simulink model "OASIS"  (R2024b)
settings: Solver=ode3  StartTime=0.0  StopTime=86400  FixedStep=1  MaxStep=0.1  RelTol=1e-3
PostLoadFcn:
  | init_OASIS
InitFcn:
  | init_OASIS
values from neighbouring files (symbols this model uses):
  DiscreteON = 1    [init_OASIS.m]
  GridON = 1    [init_OASIS.m]
  P_cargador_EV = 50000    [init_OASIS.m]
undefined symbols (not defined in the file or in its folder): DiscIntNeverNeededParam, Tamb
(part 3 of 3)

== system OASIS/Cuadro de Control 2 ==
  note: Battery
  note: Manual Mode
  note: Manual Power Ref. (kW)
  note: Power (kW)
  note: Charge
  note: Discharge
  note: State of Charge
  note: Voltage
  note: Current
  Dashboard Scope : DashboardScope  Ymin=-2000  Ymax=2000  LegendPosition=Hide  ScaleAtStop=off
  Dashboard Scope1 : DashboardScope  Ymin=0  Ymax=100  LegendPosition=Hide  ScaleAtStop=off
  Gauge : CircularGaugeBlock  LabelPosition=Hide  ScaleMax=450
  Gauge1 : CircularGaugeBlock  LabelPosition=Hide  ScaleMin=-5000  ScaleMax=5000  TickInterval=1000
  Slider : SliderBlock  LabelPosition=Hide  ScaleMin=-2000  ScaleMax=2000
  Toggle Switch : ToggleSwitchBlock  LabelPosition=Hide
      settings: Values={{'Off', 'On'}, [0 1]}

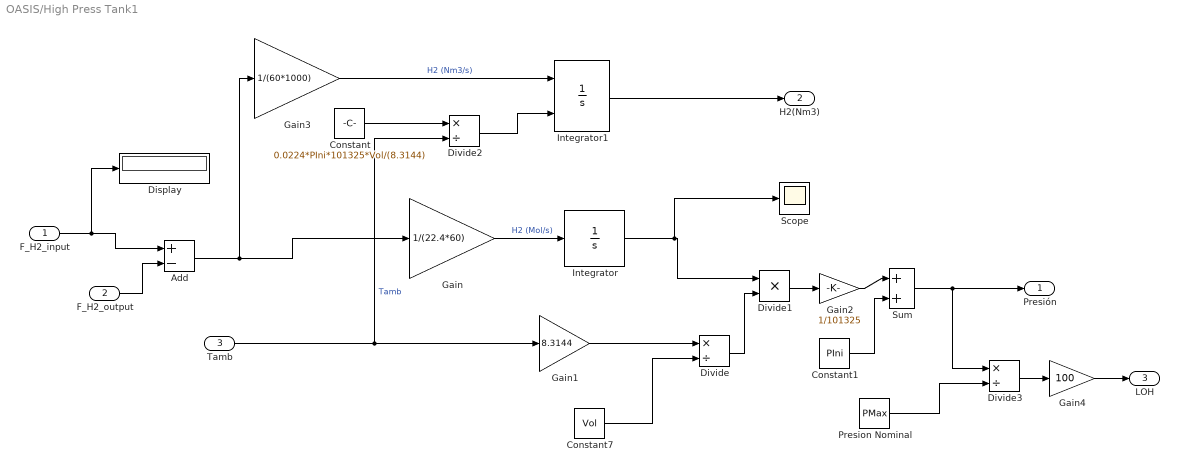
== system OASIS/High Press Tank1 ==
  F_H2_input : Inport
  F_H2_output : Inport  Port=2
  Tamb : Inport  Port=3
  Add : Sum  Inputs=+-
  Constant : Constant  Value=0.0224*PIni*101325*Vol/(8.3144)
  Constant1 : Constant  Value=PIni
  Constant7 : Constant  Value=Vol
  Display : Display
  Divide : Product  Inputs=*/
  Divide1 : Product  Inputs=**
  Divide2 : Product  Inputs=*/
  Divide3 : Product  Inputs=*/
  Gain : Gain  Gain=1/(22.4*60)
  Gain1 : Gain  Gain=8.3144
  Gain2 : Gain  Gain=1/101325
  Gain3 : Gain  Gain=1/(60*1000)
  Gain4 : Gain  Gain=100
  Integrator : Integrator
  Integrator1 : Integrator  InitialConditionSource=external  InitialCondition=PIni*101325*Vol/(8.3144*Tamb*1000)
  Presion Nominal : Constant  Value=PMax
  Scope : Scope
  Sum : Sum  Inputs=|++
  Presión : Outport
  H2(Nm3) : Outport  Port=2
  LOH : Outport  Port=3
  wires:
  Integrator/1 -> Scope/1, Divide1/1
  Divide1/1 -> Gain2/1
  Constant7/1 -> Divide/2
  Gain/1 -> Integrator/1  "H2 (Mol/s)"
  Tamb/1 -> Divide2/2, Gain1/1  "Tamb"
  Gain1/1 -> Divide/1
  Divide/1 -> Divide1/2
  Integrator1/1 -> H2(Nm3)/1
  Gain3/1 -> Integrator1/1  "H2 (Nm3/s)"
  Sum/1 -> Divide3/1, Presión/1
  Gain2/1 -> Sum/1
  Constant1/1 -> Sum/2
  Constant/1 -> Divide2/1
  Divide2/1 -> Integrator1/2
  Add/1 -> Gain3/1, Gain/1
  F_H2_input/1 -> Display/1, Add/1
  F_H2_output/1 -> Add/2
  Presion Nominal/1 -> Divide3/2
  Divide3/1 -> Gain4/1
  Gain4/1 -> LOH/1

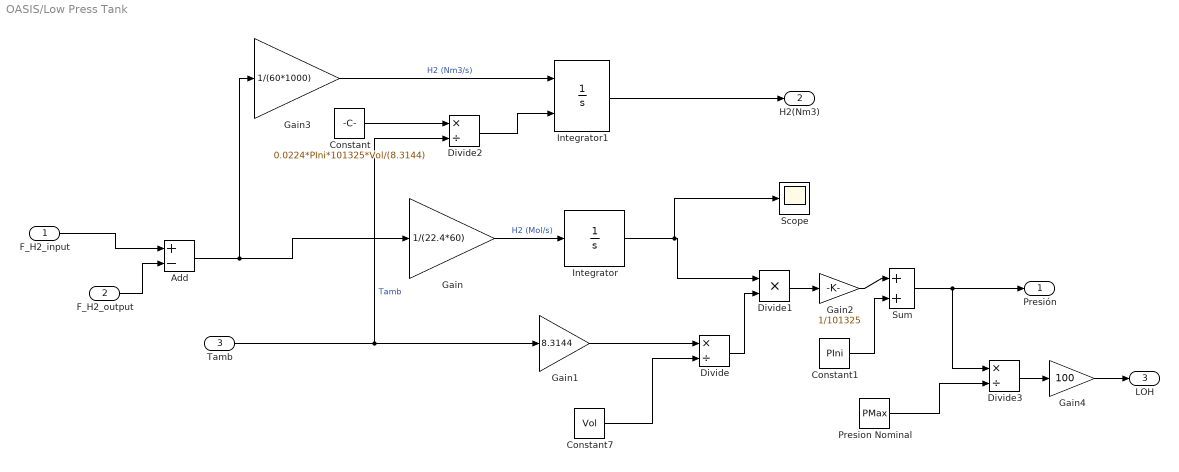
== system OASIS/Low Press Tank ==
  F_H2_input : Inport
  F_H2_output : Inport  Port=2
  Tamb : Inport  Port=3
  Add : Sum  Inputs=+-
  Constant : Constant  Value=0.0224*PIni*101325*Vol/(8.3144)
  Constant1 : Constant  Value=PIni
  Constant7 : Constant  Value=Vol
  Divide : Product  Inputs=*/
  Divide1 : Product  Inputs=**
  Divide2 : Product  Inputs=*/
  Divide3 : Product  Inputs=*/
  Gain : Gain  Gain=1/(22.4*60)
  Gain1 : Gain  Gain=8.3144
  Gain2 : Gain  Gain=1/101325
  Gain3 : Gain  Gain=1/(60*1000)
  Gain4 : Gain  Gain=100
  Integrator : Integrator
  Integrator1 : Integrator  InitialConditionSource=external  InitialCondition=PIni*101325*Vol/(8.3144*Tamb*1000)
  Presion Nominal : Constant  Value=PMax
  Scope : Scope
  Sum : Sum  Inputs=|++
  Presión : Outport
  H2(Nm3) : Outport  Port=2
  LOH : Outport  Port=3
  wires:
  Integrator/1 -> Scope/1, Divide1/1
  Divide1/1 -> Gain2/1
  Constant7/1 -> Divide/2
  Gain/1 -> Integrator/1  "H2 (Mol/s)"
  Tamb/1 -> Divide2/2, Gain1/1  "Tamb"
  Gain1/1 -> Divide/1
  Divide/1 -> Divide1/2
  Integrator1/1 -> H2(Nm3)/1
  Gain3/1 -> Integrator1/1  "H2 (Nm3/s)"
  Sum/1 -> Divide3/1, Presión/1
  Gain2/1 -> Sum/1
  Constant1/1 -> Sum/2
  Constant/1 -> Divide2/1
  Divide2/1 -> Integrator1/2
  Add/1 -> Gain3/1, Gain/1
  F_H2_input/1 -> Add/1
  F_H2_output/1 -> Add/2
  Presion Nominal/1 -> Divide3/2
  Divide3/1 -> Gain4/1
  Gain4/1 -> LOH/1

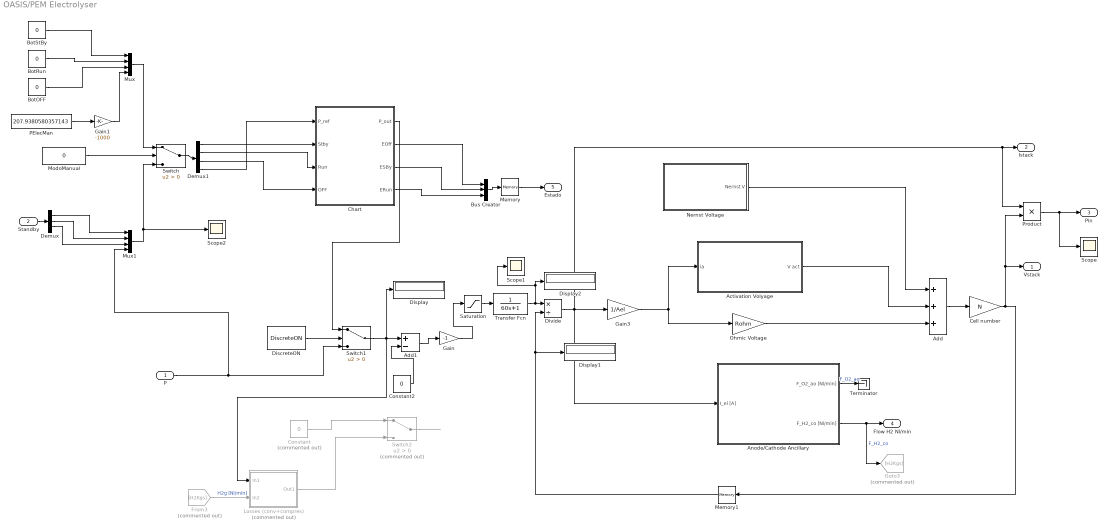
== system OASIS/PEM Electrolyser ==
  P : Inport
  Standby : Inport  Port=2
  Activation Volyage : Subsystem
  Add : Sum  Inputs=+++
  Add1 : Sum  Inputs=+-
  Anode/Cathode Ancillary : Subsystem
  BotOFF : Constant  Value=0
  BotRun : Constant  Value=0
  BotStBy : Constant  Value=0
  Bus Creator : BusCreator  Inputs=3
  Cell number : Gain  Gain=N
  Chart : Stateflow chart  TreatAsAtomicUnit=on
  Constant : Constant  Commented=on  Value=0
  Constant2 : Constant  Value=0
  Demux : Demux  Outputs=3
  Demux1 : Demux
  DiscreteON : Constant  Value=DiscreteON
  Display : Display
  Display1 : Display
  Display2 : Display
  Divide : Product  Inputs=*/
  From3 : From  Commented=on  GotoTag=H2Kgs
  Gain : Gain  Gain=-1
  Gain1 : Gain  Gain=-1000
  Gain3 : Gain  Gain=1/Ael
  Goto3 : Goto  Commented=on  GotoTag=H2Kgs
  Losses (conv+compres) : Subsystem  Commented=on
  Memory : Memory
  Memory1 : Memory  InitialCondition=115
  ModoManual : Constant  Value=0
  Mux : Mux
  Mux1 : Mux
  Nernst Voltage : Subsystem
  Ohmic Voltage : Gain  Gain=Rohm
  PElecMan : Constant  Value=207.9380580357143
  Product : Product
  Saturation : Saturate  UpperLimit=Pmax  LowerLimit=0
  Scope : Scope
  Scope1 : Scope
  Scope2 : Scope
  Switch : Switch  Criteria=u2 > Threshold  SaturateOnIntegerOverflow=off  InputSameDT=off
  Switch1 : Switch  Criteria=u2 > Threshold  SaturateOnIntegerOverflow=off  InputSameDT=off
  Switch2 : Switch  Commented=on  Criteria=u2 > Threshold  SaturateOnIntegerOverflow=off  InputSameDT=off
  Terminator : Terminator
  Transfer Fcn : TransferFcn  Denominator=[60 1]
  Vstack : Outport  VectorParamsAs1DForOutWhenUnconnected=off
  Istack : Outport  Port=2  VectorParamsAs1DForOutWhenUnconnected=off
  Pin : Outport  Port=3  VectorParamsAs1DForOutWhenUnconnected=off
  "Flow H2 Nl/min " : Outport  Port=4  VectorParamsAs1DForOutWhenUnconnected=off
  Estado : Outport  Port=5  VectorParamsAs1DForOutWhenUnconnected=off
  wires:
  Product/1 -> Scope/1, Pin/1
  Gain/1 -> Saturation/1
  Ohmic Voltage/1 -> Add/3
  Activation Volyage/1(V act) -> Add/2
  Cell number/1 -> Memory1/1, Vstack/1, Product/2
  Nernst Voltage/1(Nernst V) -> Add/1
  Add/1 -> Cell number/1
  Divide/1 -> Gain3/1, Istack/1, Product/1, Anode/Cathode Ancillary/1(I_el [A])
  Memory1/1 -> Display1/1, Divide/2
  Gain3/1 -> Ohmic Voltage/1, Activation Volyage/1(ia)
  Anode/Cathode Ancillary/2(F_H2_co [Nl/min]) -> Goto3/1, "Flow H2 Nl/min "/1  "F_H2_co"
  ModoManual/1 -> Switch/2
  PElecMan/1 -> Gain1/1
  P/1 -> Mux1/4, Switch1/3
  Chart/1(P_out) -> Switch1/1
  Saturation/1 -> Transfer Fcn/1
  Transfer Fcn/1 -> Scope1/1, Display2/1, Divide/1
  DiscreteON/1 -> Switch1/2
  Add1/1 -> Gain/1
  Switch1/1 -> Display/1, Add1/1, Losses (conv+compres)/1(In1)
  Constant/1 -> Switch2/1
  Losses (conv+compres)/1(Out1) -> Switch2/3
  From3/1 -> Losses (conv+compres)/2(In2)  "H2g [Nl/min]"
  Bus Creator/1 -> Memory/1
  Memory/1 -> Estado/1
  BotStBy/1 -> Mux/1
  BotRun/1 -> Mux/2
  BotOFF/1 -> Mux/3
  Gain1/1 -> Mux/4
  Mux/1 -> Switch/1
  Switch/1 -> Demux1/1
  Demux1/1 -> Chart/2(Stby)
  Demux1/2 -> Chart/3(Run)
  Demux1/3 -> Chart/4(OFF)
  Demux1/4 -> Chart/1(P_ref)
  Standby/1 -> Demux/1
  Demux/1 -> Mux1/1
  Demux/2 -> Mux1/2
  Mux1/1 -> Scope2/1, Switch/3
  Demux/3 -> Mux1/3
  Chart/2(EOff) -> Bus Creator/1
  Chart/3(ESBy) -> Bus Creator/2
  Chart/4(ERun) -> Bus Creator/3
  Constant2/1 -> Add1/2
  Anode/Cathode Ancillary/1(F_O2_ao [Nl/min]) -> Terminator/1  "F_O2_ao"
  Switch2/1 -> ?

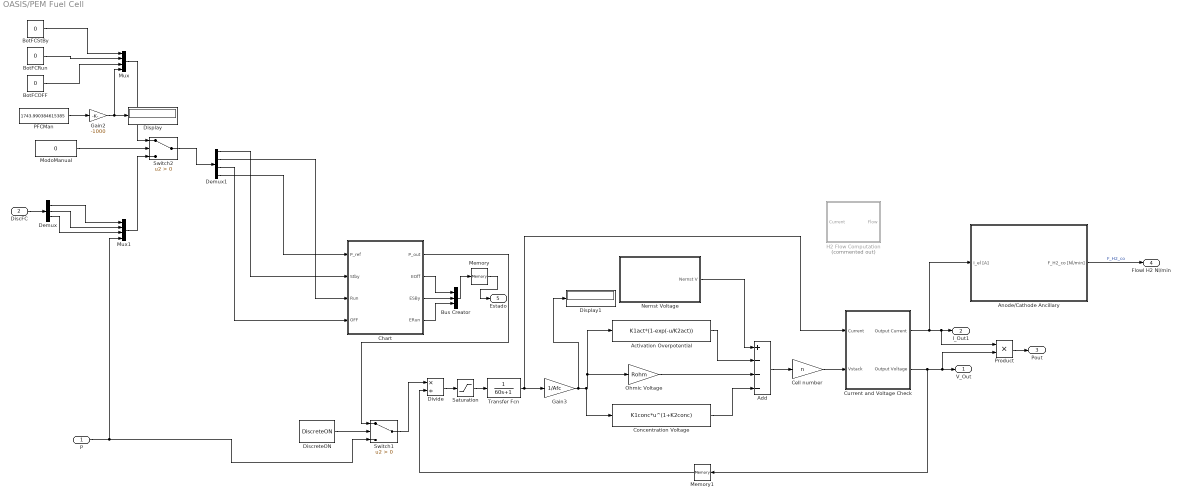
== system OASIS/PEM Fuel Cell ==
  P : Inport
  DiscFC : Inport  Port=2
  "Activation Overpotential " : Fcn  Expr=K1act*(1-exp(-u/K2act))
  Add : Sum  Inputs=+---
  Anode/Cathode Ancillary : Subsystem
  BotFCOFF : Constant  Value=0
  BotFCRun : Constant  Value=0
  BotFCStBy : Constant  Value=0
  Bus Creator : BusCreator  Inputs=3
  Cell number : Gain  Gain=n
  Chart : Stateflow chart  TreatAsAtomicUnit=on
  Concentration Voltage : Fcn  Expr=K1conc*u^(1+K2conc)
  Current and Voltage Check : Subsystem
  Demux : Demux  Outputs=3
  Demux1 : Demux
  DiscreteON : Constant  Value=DiscreteON
  Display : Display
  Display1 : Display
  Divide : Product  Inputs=*/
  Gain2 : Gain  Gain=-1000
  Gain3 : Gain  Gain=1/Afc
  H2 Flow Computation : Subsystem  Commented=on
  Memory : Memory
  Memory1 : Memory  InitialCondition=600
  ModoManual : Constant  Value=0
  Mux : Mux
  Mux1 : Mux
  Nernst Voltage : Subsystem
  Ohmic Voltage : Gain  Gain=Rohm
  PFCMan : Constant  Value=1743.990384615385
  Product : Product
  Saturation : Saturate  UpperLimit=Imax  LowerLimit=0
  Switch1 : Switch  Criteria=u2 > Threshold  SaturateOnIntegerOverflow=off  InputSameDT=off
  Switch2 : Switch  Criteria=u2 > Threshold  SaturateOnIntegerOverflow=off  InputSameDT=off
  Transfer Fcn : TransferFcn  Denominator=[60 1]
  V_Out : Outport  VectorParamsAs1DForOutWhenUnconnected=off
  I_Out1 : Outport  Port=2  VectorParamsAs1DForOutWhenUnconnected=off
  Pout : Outport  Port=3  VectorParamsAs1DForOutWhenUnconnected=off
  Flowl H2 Nl/min : Outport  Port=4  VectorParamsAs1DForOutWhenUnconnected=off
  Estado : Outport  Port=5  VectorParamsAs1DForOutWhenUnconnected=off
  wires:
  Product/1 -> Pout/1
  Cell number/1 -> Current and Voltage Check/2(Vstack)
  Divide/1 -> Saturation/1
  Current and Voltage Check/1(Output Current) -> Anode/Cathode Ancillary/1(I_el [A]), I_Out1/1, Product/1
  Current and Voltage Check/2(Output Voltage) -> V_Out/1, Product/2, Memory1/1
  "Activation Overpotential "/1 -> Add/2
  Nernst Voltage/1(Nernst V) -> Add/1
  Gain3/1 -> Display1/1, Ohmic Voltage/1, "Activation Overpotential "/1, Concentration Voltage/1
  Ohmic Voltage/1 -> Add/3
  Memory1/1 -> Divide/2
  Add/1 -> Cell number/1
  Anode/Cathode Ancillary/1(F_H2_co [Nl/min]) -> Flowl H2 Nl/min/1  "F_H2_co"
  Concentration Voltage/1 -> Add/4
  Saturation/1 -> Transfer Fcn/1
  Chart/3(ESBy) -> Bus Creator/2
  Chart/4(ERun) -> Bus Creator/3
  Chart/2(EOff) -> Bus Creator/1
  Transfer Fcn/1 -> Current and Voltage Check/1(Current), Gain3/1
  DiscreteON/1 -> Switch1/2
  Chart/1(P_out) -> Switch1/1
  Switch1/1 -> Divide/1
  Bus Creator/1 -> Memory/1
  Demux/3 -> Mux1/3
  DiscFC/1 -> Demux/1
  BotFCRun/1 -> Mux/2
  Demux/2 -> Mux1/2
  Demux/1 -> Mux1/1
  BotFCOFF/1 -> Mux/3
  Gain2/1 -> Mux/4, Display/1
  P/1 -> Switch1/3, Mux1/4
  ModoManual/1 -> Switch2/2
  Mux/1 -> Switch2/1
  BotFCStBy/1 -> Mux/1
  Mux1/1 -> Switch2/3
  PFCMan/1 -> Gain2/1
  Switch2/1 -> Demux1/1
  Memory/1 -> Estado/1
  Demux1/4 -> Chart/1(P_ref)
  Demux1/1 -> Chart/2(Stby)
  Demux1/2 -> Chart/3(Run)
  Demux1/3 -> Chart/4(OFF)

== system OASIS/Predicciones LSTM ==
  Clock1 : Clock
  From Workspace1 : FromWorkspace  VariableName=features_solar  SampleTime=900
  From Workspace2 : FromWorkspace  VariableName=dia_anno  SampleTime=1
  From Workspace3 : FromWorkspace  VariableName=features_precio  SampleTime=1
  From Workspace4 : FromWorkspace  VariableName=dia_semana  SampleTime=1
  Gain4 : Gain  Gain=490
  Modelo LSTM Irradianza : M-S-Function  FunctionName=lstm_sol
  Modelo LSTM Precio : M-S-Function  FunctionName=lstm_precios
  W : Outport
  €/MW : Outport  Port=2
  W/m2 : Outport  Port=3
  wires:
  Clock1/1 -> Modelo LSTM Precio/2, Modelo LSTM Irradianza/2
  Gain4/1 -> W/1  "W"
  Modelo LSTM Precio/1 -> €/MW/1  "€/MW"
  From Workspace3/1 -> Modelo LSTM Precio/1
  Modelo LSTM Irradianza/1 -> W/m2/1, Gain4/1  "W/m2"
  From Workspace1/1 -> Modelo LSTM Irradianza/1
  From Workspace2/1 -> Modelo LSTM Precio/3
  From Workspace4/1 -> Modelo LSTM Precio/4

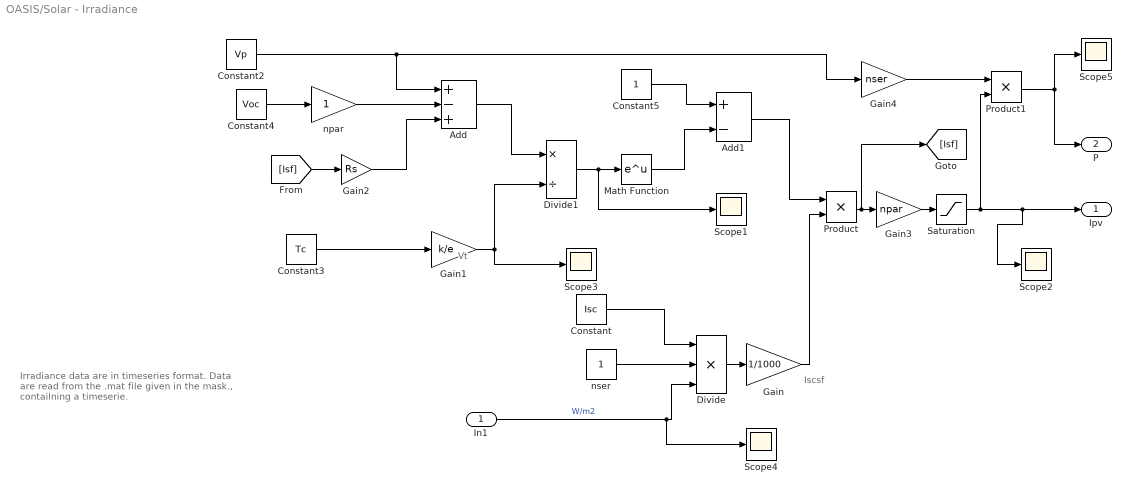
== system OASIS/Solar - Irradiance ==
  note: Vt
  note: Iscsf
  note: Irradiance data are in timeseries format.
      |
      | Data are read from the .mat file given in the mask., contailning a timeserie.
  In1 : Inport
  Add : Sum  Inputs=+-+
  Add1 : Sum  Inputs=+-
  Constant : Constant  Value=Isc
  Constant2 : Constant  Value=Vp
  Constant3 : Constant  Value=Tc
  Constant4 : Constant  Value=Voc
  Constant5 : Constant
  Divide : Product  Inputs=***
  Divide1 : Product  Inputs=*/
  Gain : Gain  Gain=1/1000
  Gain1 : Gain  Gain=k/e
  Gain2 : Gain  Gain=Rs
  Gain3 : Gain  Gain=npar
  Gain4 : Gain  Gain=nser
  Math Function : Math  SignedPower=on
  Product : Product
  Product1 : Product
  Saturation : Saturate  UpperLimit=inf  LowerLimit=0
  Scope{1..5} (5 alike) : Scope
  npar : Gain
  nser : Constant
  Ipv : Outport  VectorParamsAs1DForOutWhenUnconnected=off
  P : Outport  Port=2  VectorParamsAs1DForOutWhenUnconnected=off
  wires:
  Constant/1 -> Divide/1
  nser/1 -> Divide/2
  Divide/1 -> Gain/1
  Gain/1 -> Product/2
  Gain1/1 -> Scope3/1, Divide1/2
  Constant2/1 -> Gain4/1, Add/1
  Constant4/1 -> npar/1
  [Isf] -> Gain2/1
  Gain2/1 -> Add/3
  Divide1/1 -> Scope1/1, Math Function/1
  Math Function/1 -> Add1/2
  Constant5/1 -> Add1/1
  Add1/1 -> Product/1
  Add/1 -> Divide1/1
  Saturation/1 -> Product1/2, Scope2/1, Ipv/1
  Constant3/1 -> Gain1/1
  npar/1 -> Add/2
  Product1/1 -> Scope5/1, P/1
  In1/1 -> Scope4/1, Divide/3  "W/m2"
  Gain4/1 -> Product1/1
  Product/1 -> [Isf], Gain3/1
  Gain3/1 -> Saturation/1

== system OASIS/Subsystem2 ==

== system OASIS/Subsystem3 ==

== system OASIS/Battery/Charge ==
  Intensidad : Inport
  IntegralI : Inport  Port=2
  Fcn1 : Fcn  Expr=Kbt*C120bt/(C120bt+0.1*u)
  Product : Product
  Out1 : Outport  VectorParamsAs1DForOutWhenUnconnected=off
  wires:
  Fcn1/1 -> Product/2
  Product/1 -> Out1/1
  Intensidad/1 -> Product/1
  IntegralI/1 -> Fcn1/1

== system OASIS/Battery/Discharge ==
  Intensidad : Inport
  IntegralI : Inport  Port=2
  Fcn1 : Fcn  Expr=Kbt*C120bt/((C120bt-u))
  Product : Product
  Out1 : Outport  VectorParamsAs1DForOutWhenUnconnected=off
  wires:
  Intensidad/1 -> Product/1
  Product/1 -> Out1/1
  Fcn1/1 -> Product/2
  IntegralI/1 -> Fcn1/1

== system OASIS/Battery/SOC Computation ==
  In1 : Inport
  Add3 : Sum  Inputs=+-
  C120,bt2 : Constant  Value=C120bt
  Divide2 : Product  Inputs=/*
  Gain6 : Gain  Gain=100
  Out1 : Outport  VectorParamsAs1DForOutWhenUnconnected=off
  wires:
  Add3/1 -> Gain6/1
  In1/1 -> Add3/2
  Gain6/1 -> Divide2/2
  C120,bt2/1 -> Divide2/1, Add3/1
  Divide2/1 -> Out1/1

== system OASIS/Battery/SOC=100 or SOC=0 ==
  ISOC : Inport
  P : Inport  Port=2
  Constant : Constant  Value=100
  Constant1 : Constant  Value=0
  Constant2 : Constant  Value=0
  Gain2 : Gain  Gain=-1
  Logical Operator : Logic  AllPortsSameDT=off  OutDataTypeStr=boolean
  Logical Operator1 : Logic  Operator=OR  AllPortsSameDT=off  OutDataTypeStr=boolean
  Product : Product
  Relational Operator : RelationalOperator  OutDataTypeStr=boolean  InputSameDT=off
  Relational Operator1 : RelationalOperator  Operator=<=  OutDataTypeStr=boolean  InputSameDT=off
  Relational Operator2 : RelationalOperator  OutDataTypeStr=boolean  InputSameDT=off
  Sign : Signum
  Out1 : Outport  VectorParamsAs1DForOutWhenUnconnected=off
  wires:
  P/1 -> Sign/1
  Sign/1 -> Relational Operator2/1, Product/2
  ISOC/1 -> Relational Operator1/1, Product/1
  Product/1 -> Gain2/1
  Gain2/1 -> Relational Operator/1
  Constant/1 -> Relational Operator/2
  Constant1/1 -> Relational Operator1/2
  Constant2/1 -> Relational Operator2/2
  Relational Operator2/1 -> Logical Operator/1
  Relational Operator1/1 -> Logical Operator/2
  Logical Operator1/1 -> Out1/1
  Relational Operator/1 -> Logical Operator1/1
  Logical Operator/1 -> Logical Operator1/2

== system OASIS/PEM Electrolyser/Activation Volyage ==
  ia : Inport
  Add1 : Sum
  Gain : Gain  Gain=R*Tel/F
  Gain1 : Gain  Gain=0.5/iao
  Gain2 : Gain  Gain=0.5/ico
  "asinh " : Fcn  Expr=log(u+sqrt(u*u+1))
  asinh 1 : Fcn  Expr=log(u+sqrt(u*u+1))
  V act : Outport  VectorParamsAs1DForOutWhenUnconnected=off
  wires:
  Gain1/1 -> "asinh "/1
  ia/1 -> Gain2/1, Gain1/1
  Gain/1 -> V act/1
  Gain2/1 -> asinh 1/1
  asinh 1/1 -> Add1/2
  "asinh "/1 -> Add1/1
  Add1/1 -> Gain/1

== system OASIS/PEM Electrolyser/Anode//Cathode Ancillary ==
  I_el [A] : Inport
  4F : Constant  Value=4*F
  Display1 : Display
  Divide1 : Product  Inputs=*/
  Gain : Gain  Gain=2
  Gain2 : Gain  Gain=22.4*60
  Gain4 : Gain  Gain=0.0899/60
  Scope1 : Scope  NumInputPorts=2
  n : Gain  Gain=N
  F_O2_ao [Nl/min] : Outport
  F_H2_co [Nl/min] : Outport  Port=2
  wires:
  4F/1 -> Divide1/2  "4F"
  Gain/1 -> Gain4/1, Scope1/2, F_H2_co [Nl/min]/1  "H2g [Nl/min]"
  Gain2/1 -> Scope1/1, F_O2_ao [Nl/min]/1, Gain/1  "O2g [Nl/min]"
  Divide1/1 -> Gain2/1  "O2g [mol/s]"
  n/1 -> Divide1/1  "n"
  I_el [A]/1 -> n/1  "I_el"
  Gain4/1 -> Display1/1  "kg/s]"

== system OASIS/PEM Electrolyser/Chart/CRampa ==
  Ref : Inport  OutDataTypeStr=double  PortDimensions=1
  Reset : Inport  Port=2  OutDataTypeStr=double  PortDimensions=1
  f : TriggerPort  TriggerType=function-call  VariantControl=(inherit)
      settings: CopyFcn=Stateflow.SLINSF.SimulinkMan.removeBlockPreDeleteFcn  PreDeleteFcn=Stateflow.SLINSF.SimulinkMan.unsafePredeleteFcn
  Constant : Constant  Value=180
  Discrete-Time Integrator : DiscreteIntegrator  ExternalReset=level  SampleTime=-1  ICPrevOutput=DiscIntNeverNeededParam  ICPrevScaledInput=DiscIntNeverNeededParam
  Divide : Product  Inputs=/*
  Gain : Gain
  PSal : Outport
  wires:
  Ref/1 -> Divide/2
  Discrete-Time Integrator/1 -> PSal/1
  Divide/1 -> Gain/1
  Gain/1 -> Discrete-Time Integrator/1
  Constant/1 -> Divide/1
  Reset/1 -> Discrete-Time Integrator/2

== system OASIS/PEM Electrolyser/Chart/EOFF1 ==
  P_ref : Inport
  Stby : Inport  Port=2
  Action Port : ActionPort
      settings: CopyFcn=Stateflow.SLINSF.SimulinkMan.removeBlockPreDeleteFcn  PreDeleteFcn=Stateflow.SLINSF.SimulinkMan.unsafePredeleteFcn
  Constant : Constant  Value=0
  Constant1 : Constant
  Constant2 : Constant  Value=0
  Constant3 : Constant  Value=0
  P_out : Outport
  EOff : Outport  Port=2
  ESBy : Outport  Port=3
  ERun : Outport  Port=4
  wires:
  Constant/1 -> P_out/1
  Constant3/1 -> ERun/1
  Constant2/1 -> ESBy/1
  Constant1/1 -> EOff/1

== system OASIS/PEM Electrolyser/Chart/Run1 ==
  P_ref : Inport
  Stby : Inport  Port=2
  Action Port : ActionPort
      settings: CopyFcn=Stateflow.SLINSF.SimulinkMan.removeBlockPreDeleteFcn  PreDeleteFcn=Stateflow.SLINSF.SimulinkMan.unsafePredeleteFcn
  Constant2 : Constant  Value=0
  Constant3 : Constant  Value=0
  Constant4 : Constant
  P_out : Outport
  EOff : Outport  Port=2
  ESBy : Outport  Port=3
  ERun : Outport  Port=4
  wires:
  P_ref/1 -> P_out/1
  Constant3/1 -> ESBy/1
  Constant2/1 -> EOff/1
  Constant4/1 -> ERun/1

== system OASIS/PEM Electrolyser/Chart/StandBy ==
  P_ref : Inport
  Stby : Inport  Port=2
  Run : Inport  Port=3
  Action Port : ActionPort
      settings: CopyFcn=Stateflow.SLINSF.SimulinkMan.removeBlockPreDeleteFcn  PreDeleteFcn=Stateflow.SLINSF.SimulinkMan.unsafePredeleteFcn
  Constant1 : Constant  Value=0
  Constant2 : Constant  Value=0
  Constant3 : Constant
  Constant4 : Constant  Value=0
  P_out : Outport
  EOff : Outport  Port=2
  ESBy : Outport  Port=3
  ERun : Outport  Port=4
  wires:
  Constant3/1 -> ESBy/1
  Constant4/1 -> ERun/1
  Constant2/1 -> EOff/1
  Constant1/1 -> P_out/1

== system OASIS/PEM Electrolyser/Chart/Trans1 ==
  P_ref : Inport
  Stby : Inport  Port=2
  Action Port : ActionPort
      settings: CopyFcn=Stateflow.SLINSF.SimulinkMan.removeBlockPreDeleteFcn  PreDeleteFcn=Stateflow.SLINSF.SimulinkMan.unsafePredeleteFcn
  Constant : Constant  Value=0
  Constant2 : Constant
  Constant3 : Constant
  Constant4 : Constant  Value=0
  P_out : Outport
  EOff : Outport  Port=2
  ESBy : Outport  Port=3
  ERun : Outport  Port=4
  wires:
  Constant/1 -> P_out/1
  Constant3/1 -> ESBy/1
  Constant4/1 -> ERun/1
  Constant2/1 -> EOff/1

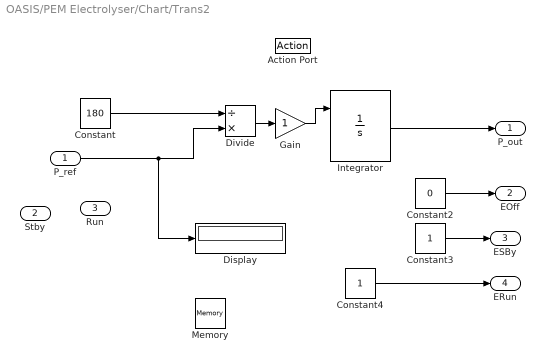
== system OASIS/PEM Electrolyser/Chart/Trans2 ==
  P_ref : Inport
  Stby : Inport  Port=2
  Run : Inport  Port=3
  Action Port : ActionPort
      settings: CopyFcn=Stateflow.SLINSF.SimulinkMan.removeBlockPreDeleteFcn  PreDeleteFcn=Stateflow.SLINSF.SimulinkMan.unsafePredeleteFcn
  Constant : Constant  Value=180
  Constant2 : Constant  Value=0
  Constant3 : Constant
  Constant4 : Constant
  Display : Display
  Divide : Product  Inputs=/*
  Gain : Gain
  Integrator : Integrator  ExternalReset=rising  LimitOutput=on  UpperSaturationLimit=0
  Memory : Memory
  P_out : Outport
  EOff : Outport  Port=2
  ESBy : Outport  Port=3
  ERun : Outport  Port=4
  wires:
  Constant/1 -> Divide/1
  Integrator/1 -> P_out/1
  P_ref/1 -> Display/1, Divide/2
  Divide/1 -> Gain/1
  Gain/1 -> Integrator/1
  Constant3/1 -> ESBy/1
  Constant4/1 -> ERun/1
  Constant2/1 -> EOff/1

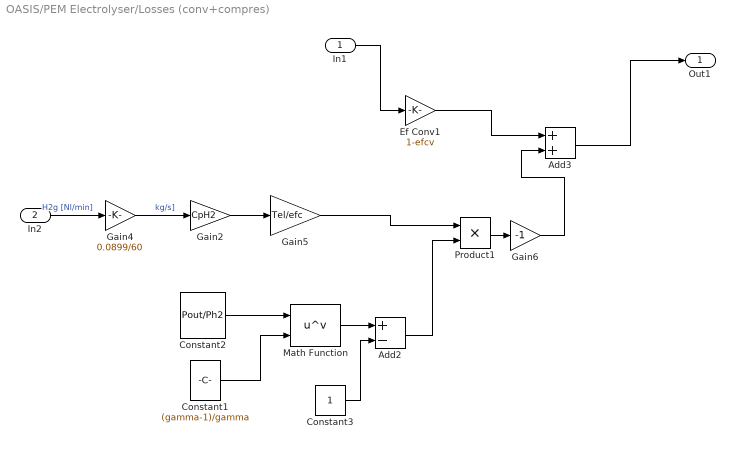
== system OASIS/PEM Electrolyser/Losses (conv+compres) ==
  In1 : Inport
  In2 : Inport  Port=2
  Add2 : Sum  Inputs=+-
  Add3 : Sum
  Constant1 : Constant  Value=(gamma-1)/gamma
  Constant2 : Constant  Value=Pout/Ph2
  Constant3 : Constant
  Ef Conv1 : Gain  Gain=1-efcv
  Gain2 : Gain  Gain=CpH2
  Gain4 : Gain  Gain=0.0899/60
  Gain5 : Gain  Gain=Tel/efc
  Gain6 : Gain  Gain=-1
  Math Function : Math  Operator=pow
  Product1 : Product
  Out1 : Outport
  wires:
  Ef Conv1/1 -> Add3/1
  In2/1 -> Gain4/1  "H2g [Nl/min]"
  Gain4/1 -> Gain2/1  "kg/s]"
  Gain2/1 -> Gain5/1
  Constant3/1 -> Add2/2
  Constant2/1 -> Math Function/1
  Gain5/1 -> Product1/1
  Constant1/1 -> Math Function/2
  Gain6/1 -> Add3/2
  Product1/1 -> Gain6/1
  Math Function/1 -> Add2/1
  Add2/1 -> Product1/2
  In1/1 -> Ef Conv1/1
  Add3/1 -> Out1/1

== system OASIS/PEM Electrolyser/Nernst Voltage ==
  Add1 : Sum  Inputs=+-
  Add2 : Sum  Inputs=+++
  Constant : Constant  Value=E0
  K1n : Gain  Gain=K1n
  K2n : Gain  Gain=2.3*R*log(Ph2*Ph2*Po2)/(4*F)
  Scope : Scope
  Scope1 : Scope
  Scope2 : Scope
  T el : Constant  Value=Tel
  T0 El : Constant  Value=298
  Nernst V : Outport  VectorParamsAs1DForOutWhenUnconnected=off
  wires:
  K2n/1 -> Add2/2, Scope1/1
  K1n/1 -> Add2/3
  T el/1 -> Add1/1, K2n/1
  Add2/1 -> Nernst V/1, Scope2/1
  Add1/1 -> K1n/1
  T0 El/1 -> Add1/2
  Constant/1 -> Add2/1, Scope/1

== system OASIS/PEM Fuel Cell/Anode//Cathode Ancillary ==
  I_el [A] : Inport
  4F : Constant  Value=4*F
  Divide1 : Product  Inputs=*/
  Gain : Gain  Gain=2
  Gain2 : Gain  Gain=22.4*60
  n : Gain  Gain=n
  F_H2_co [Nl/min] : Outport
  wires:
  4F/1 -> Divide1/2  "4F"
  Gain/1 -> F_H2_co [Nl/min]/1  "H2g [Nl/min]"
  Gain2/1 -> Gain/1  "O2g [Nl/min]"
  Divide1/1 -> Gain2/1  "O2g [mol/s]"
  n/1 -> Divide1/1  "n"
  I_el [A]/1 -> n/1  "I_el"

== system OASIS/PEM Fuel Cell/Chart/CRampa ==
  Ref : Inport  OutDataTypeStr=double  PortDimensions=1
  Reset : Inport  Port=2  OutDataTypeStr=double  PortDimensions=1
  f : TriggerPort  TriggerType=function-call  VariantControl=(inherit)
      settings: CopyFcn=Stateflow.SLINSF.SimulinkMan.removeBlockPreDeleteFcn  PreDeleteFcn=Stateflow.SLINSF.SimulinkMan.unsafePredeleteFcn
  Constant : Constant  Value=180
  Discrete-Time Integrator : DiscreteIntegrator  ExternalReset=level  SampleTime=-1  ICPrevOutput=DiscIntNeverNeededParam  ICPrevScaledInput=DiscIntNeverNeededParam
  Divide : Product  Inputs=/*
  Gain : Gain
  PSal : Outport
  wires:
  Ref/1 -> Divide/2
  Discrete-Time Integrator/1 -> PSal/1
  Divide/1 -> Gain/1
  Gain/1 -> Discrete-Time Integrator/1
  Constant/1 -> Divide/1
  Reset/1 -> Discrete-Time Integrator/2

== system OASIS/PEM Fuel Cell/Chart/EOFF1 ==
  P_ref : Inport
  Stby : Inport  Port=2
  Action Port : ActionPort
      settings: CopyFcn=Stateflow.SLINSF.SimulinkMan.removeBlockPreDeleteFcn  PreDeleteFcn=Stateflow.SLINSF.SimulinkMan.unsafePredeleteFcn
  Constant : Constant  Value=0
  Constant1 : Constant
  Constant2 : Constant  Value=0
  Constant3 : Constant  Value=0
  P_out : Outport
  EOff : Outport  Port=2
  ESBy : Outport  Port=3
  ERun : Outport  Port=4
  wires:
  Constant/1 -> P_out/1
  Constant3/1 -> ERun/1
  Constant2/1 -> ESBy/1
  Constant1/1 -> EOff/1

== system OASIS/PEM Fuel Cell/Chart/Run1 ==
  P_ref : Inport
  Stby : Inport  Port=2
  Action Port : ActionPort
      settings: CopyFcn=Stateflow.SLINSF.SimulinkMan.removeBlockPreDeleteFcn  PreDeleteFcn=Stateflow.SLINSF.SimulinkMan.unsafePredeleteFcn
  Constant2 : Constant  Value=0
  Constant3 : Constant  Value=0
  Constant4 : Constant
  P_out : Outport
  EOff : Outport  Port=2
  ESBy : Outport  Port=3
  ERun : Outport  Port=4
  wires:
  P_ref/1 -> P_out/1
  Constant3/1 -> ESBy/1
  Constant2/1 -> EOff/1
  Constant4/1 -> ERun/1

== system OASIS/PEM Fuel Cell/Chart/StandBy ==
  P_ref : Inport
  Stby : Inport  Port=2
  Run : Inport  Port=3
  Action Port : ActionPort
      settings: CopyFcn=Stateflow.SLINSF.SimulinkMan.removeBlockPreDeleteFcn  PreDeleteFcn=Stateflow.SLINSF.SimulinkMan.unsafePredeleteFcn
  Constant1 : Constant  Value=0
  Constant2 : Constant  Value=0
  Constant3 : Constant
  Constant4 : Constant  Value=0
  P_out : Outport
  EOff : Outport  Port=2
  ESBy : Outport  Port=3
  ERun : Outport  Port=4
  wires:
  Constant3/1 -> ESBy/1
  Constant4/1 -> ERun/1
  Constant2/1 -> EOff/1
  Constant1/1 -> P_out/1

== system OASIS/PEM Fuel Cell/Chart/Trans1 ==
  P_ref : Inport
  Stby : Inport  Port=2
  Action Port : ActionPort
      settings: CopyFcn=Stateflow.SLINSF.SimulinkMan.removeBlockPreDeleteFcn  PreDeleteFcn=Stateflow.SLINSF.SimulinkMan.unsafePredeleteFcn
  Constant : Constant  Value=0
  Constant2 : Constant
  Constant3 : Constant
  Constant4 : Constant  Value=0
  P_out : Outport
  EOff : Outport  Port=2
  ESBy : Outport  Port=3
  ERun : Outport  Port=4
  wires:
  Constant/1 -> P_out/1
  Constant3/1 -> ESBy/1
  Constant4/1 -> ERun/1
  Constant2/1 -> EOff/1

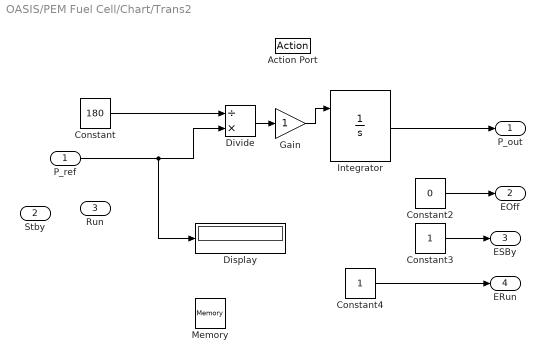
== system OASIS/PEM Fuel Cell/Chart/Trans2 ==
  P_ref : Inport
  Stby : Inport  Port=2
  Run : Inport  Port=3
  Action Port : ActionPort
      settings: CopyFcn=Stateflow.SLINSF.SimulinkMan.removeBlockPreDeleteFcn  PreDeleteFcn=Stateflow.SLINSF.SimulinkMan.unsafePredeleteFcn
  Constant : Constant  Value=180
  Constant2 : Constant  Value=0
  Constant3 : Constant
  Constant4 : Constant
  Display : Display
  Divide : Product  Inputs=/*
  Gain : Gain
  Integrator : Integrator  ExternalReset=rising  LimitOutput=on  UpperSaturationLimit=0
  Memory : Memory
  P_out : Outport
  EOff : Outport  Port=2
  ESBy : Outport  Port=3
  ERun : Outport  Port=4
  wires:
  Constant/1 -> Divide/1
  Integrator/1 -> P_out/1
  P_ref/1 -> Display/1, Divide/2
  Divide/1 -> Gain/1
  Gain/1 -> Integrator/1
  Constant3/1 -> ESBy/1
  Constant4/1 -> ERun/1
  Constant2/1 -> EOff/1

== system OASIS/PEM Fuel Cell/Current and Voltage Check ==
  Current : Inport
  Vstack : Inport  Port=2
  Constant5 : Constant  Value=0.5
  Constant6 : Constant  Value=0
  Display : Display
  Display1 : Display
  Switch : Switch  Criteria=u2 > Threshold  SaturateOnIntegerOverflow=off  InputSameDT=off
  Switch1 : Switch  Criteria=u2 > Threshold  SaturateOnIntegerOverflow=off  InputSameDT=off
  Output Current : Outport  VectorParamsAs1DForOutWhenUnconnected=off
  Output Voltage : Outport  Port=2  VectorParamsAs1DForOutWhenUnconnected=off
  wires:
  Switch/1 -> Output Voltage/1
  Constant5/1 -> Switch/3
  Switch1/1 -> Output Current/1
  Constant6/1 -> Switch1/3
  Current/1 -> Display/1, Switch1/1
  Vstack/1 -> Display1/1, Switch/2, Switch/1, Switch1/2

== system OASIS/PEM Fuel Cell/H2 Flow Computation ==
  Current : Inport
  Cell number1 : Gain  Gain=n
  Convertion : Gain  Gain=2/1000
  Divide2 : Product  Inputs=*/
  Faraday*2 : Constant  Value=2*96485.33289
  Flow : Outport  VectorParamsAs1DForOutWhenUnconnected=off
  wires:
  Cell number1/1 -> Divide2/1
  Divide2/1 -> Convertion/1
  Convertion/1 -> Flow/1
  Current/1 -> Cell number1/1
  Faraday*2/1 -> Divide2/2

== system OASIS/PEM Fuel Cell/Nernst Voltage ==
  Add1 : Sum  Inputs=+-
  Add2 : Sum
  Constant : Constant  Value=u0
  Gain : Gain  Gain=K1t
  T FC : Constant  Value=Tst
  T0 FC : Constant  Value=T0st
  Nernst V : Outport  VectorParamsAs1DForOutWhenUnconnected=off
  wires:
  T FC/1 -> Add1/1
  Add2/1 -> Nernst V/1
  Add1/1 -> Gain/1
  T0 FC/1 -> Add1/2
  Constant/1 -> Add2/1
  Gain/1 -> Add2/2

== matlab function OASIS/Compresor/MATLAB Function ==
  data: PEnt input; Caudal output; PSalida input; PCompresor input
function Caudal = fcn(PEnt, PSalida, PCompresor)
    k = 1.4;  
    R = 4124; 
    T = 298;  
    Constante = (k-1)/k;
    
    PEnt_safe = max(PEnt, 0.001);
    PSalida_safe = max(PSalida, 0.001);
    
    % Calculamos la relación real
    Relacion = PSalida_safe / PEnt_safe;
    
    if Relacion < 1.05
        % ESCUDO 3: Cruce de presiones
        % Si el tanque destino tiene menos presión o casi la misma que el origen,
        % la ecuación diverge. Asignamos un flujo nominal seguro (ej. 10 gramos/s)
        % para que las presiones se igualen suavemente sin colapsar las matemáticas.
        Caudal = 0.01; 
    else
        % Ecuación termodinámica normal
        Den = R * T * ((Relacion^Constante) - 1);
        Caudal = Constante * PCompresor / Den;
    end
end

== stateflow chart OASIS/PEM Electrolyser/Chart ==
  settings: initializeOutput=1
  state EOFF1 [commented out]
  state Trans1 [commented out]
  state StandBy [commented out]
  state Trans2 [commented out]
  state Run [commented out]
  state Standby
    P_out=CRampa(P_ref,1);
    P_out=0;
    EOff=0;
    ESBy=1;
    ERun=0;
  state EOFF
    P_out=0;
    EOff=1;
    ESBy=0;
    ERun=0;
  state Trans3
    P_out=0;
    EOff=1;
    ESBy=1;
    ERun=0;
  state Trans4
    P_out=CRampa(P_ref,0);
    EOff=0;
    ESBy=1;
    ERun=1;
  state Run1
    P_out=P_ref;
    EOff=0;
    ESBy=0;
    ERun=1;
  state PSal = CRampa(Ref,Reset) [function]
  (default) -> EOFF1 [commented out]
  Trans2 -> Run [commented out] : after(180,sec)
  EOFF1 -> Trans1 [commented out] : [Stby==1]
  StandBy -> Trans2 [commented out] : [Run==1]
  Trans1 -> StandBy [commented out] : after(380,sec)
  Run -> StandBy [commented out] : [Stby==1]
  (default) -> EOFF
  EOFF -> Trans3 : [Stby==1]
  Trans3 -> Standby : after(380,sec)
  Standby -> Trans4 [order 1] : [Run==1]
  Trans4 -> Run1 : after(180,sec)
  Standby -> EOFF [order 2] : [OFF==1]
  Run1 -> Standby : [Stby==1]
  data: sf_internal_action_state_placeholder_data local double size=1 =0; sf_internal_action_state_placeholder_data local double size=1 =0; sf_internal_action_state_placeholder_data local double size=1 =0; sf_internal_action_state_placeholder_data local double size=1 =0; sf_internal_action_state_placeholder_data local double size=1 =0; Ref function_input double size=1; PSal function_output; Reset function_input double size=1; P_ref input; P_out output; Stby input; EOff output; ESBy output; ERun output; Run input; OFF input

== matlab function OASIS/MATLAB Function ==
  settings: updateMethod=DISCRETE
  data: Carga input; PV input; EstEl input; EstFC input; LOH input; LOH_High input; Precio input; DemandaH2 input; RefFC output; RefEl output; RefBat output; DiscEl output size=[1 3]; DiscFC output size=[1 3]; Compresor output size=1; SOC input; PVPred input; PrecioPred input
function [RefFC, RefEl, RefBat, DiscEl, DiscFC, Compresor] = fcn( ...
    Carga, PV, EstEl, EstFC, LOH, LOH_High, Precio, DemandaH2, SOC, PVPred, PrecioPred)
%#codegen
% EMS Version B'' (Version B en la memoria): A + dos ganchos con prevision.
%   Gancho 1 (PVPred): si se anticipa caida del excedente en las proximas
%       N_PV_H horas, el reparto del excedente se desplaza hacia el
%       electrolizador; si se anticipa subida, hacia la bateria.
%   Gancho 2 (PrecioPred): arbitraje de bateria dimensionado. Se busca la punta
%       de precio en N_ARB_H horas; si el beneficio neto tras perdidas supera
%       MARGEN_ARB, se compra la energia que falta para llegar a SOC_OBJ_ARB
%       repartida entre las horas hasta la punta. El electrolizador no compra
%       red por esta via.
% Todo lo demas es identico a A. Misma firma que el bloque de OASIS.slx.
% Las S-Functions entregan la senal combinada con su linea base, no la cruda.

%% Parametros (identicos a A)
PmaxBat = 1.9e6;
PmaxEl  = 2e5;
PmaxFC  = 1.3e5;
PmaxComp= 15000;

SOC_MAX_PV   = 90;
SOC_MIN_DESC = 20;
SOC_LOW      = 40;
SOC_HIGH     = 80;
SOC          = max(0, min(100, SOC));

LOH_min      = 55;
LOH_maxEL    = 95;
LOH_reserva  = 68;

LOH_High_hi     = 97;
LOH_High_lo_on  = 76;
LOH_High_lo_off = 79;
LOH_High_crit   = 72;

kWh_EL_kg   = 50;
kWh_COMP_kg = 3.6;
H2_PRECIO_EXT_KG = 8;      % EUR/kg, coste de reposicion (camion + compresion). Umbral = 149 EUR/MWh
C_comp_kg   = Precio * (kWh_COMP_kg / 1000);
C_ELcomp_kg = Precio * ((kWh_EL_kg + kWh_COMP_kg) / 1000);

TMF_s   = 2 * 3600;
Ts_s    = 1;
P_EL_min_keep = 0.20 * PmaxEl;
P_FC_min_keep = 0.25 * PmaxFC;
thr_EL     = 0.15 * PmaxEl;
FC_thr_on  = 0.08 * PmaxFC;
FC_thr_off = 0.04 * PmaxFC;
DEB_on_s  = 30;
DEB_off_s = 90;

%% Parametros de los ganchos
N_PV_H       = 2;     % horas de PVPred promediadas (tramo con skill positivo)
N_PRECIO_H   = 2;     % horas de PrecioPred promediadas para 'precio_sube'
DELTA_W_MAX  = 0.15;  % desplazamiento maximo del reparto por prevision PV
MARGEN_PRECIO= 25;    % EUR/MWh de subida prevista para 'precio_sube' (> MAE de la prevision)
CAP_BAT_kWh  = 1000;  % capacidad util de la bateria
ETA_BAT      = 0.90;  % rendimiento ida y vuelta
N_ARB_H      = 12;    % horizonte de busqueda de la punta de precio (h)
MARGEN_ARB   = 25;    % EUR/MWh de beneficio neto exigido para comprar red
SOC_OBJ_ARB  = 85;    % SOC objetivo del arbitraje, por debajo de SOC_MAX_PV

%% Estados persistentes (TMF)
persistent EL_on EL_t EL_deb FC_on FC_t FC_deb_on FC_deb_off
if isempty(EL_on), EL_on = false; EL_t = 0; EL_deb = 0; end
if isempty(FC_on), FC_on = false; FC_t = 0; FC_deb_on = 0; FC_deb_off = 0; end

%% Previsiones de corto plazo
n_pv = min(N_PV_H, numel(PVPred));
PV_near = mean(PVPred(1:max(1,n_pv)));
pv_trend = PV_near - PV;            % >0 mas excedente proximo, <0 caida

n_pr = min(N_PRECIO_H, numel(PrecioPred));
Precio_near = mean(PrecioPred(1:max(1,n_pr)));
precio_sube = (Precio_near - Precio) > MARGEN_PRECIO;

% punta de precio prevista y test economico del arbitraje
n_arb   = min(N_ARB_H, numel(PrecioPred));
p_punta = Precio;
h_punta = 0;
for k_arb = 1:n_arb
    if PrecioPred(k_arb) > p_punta
        p_punta = PrecioPred(k_arb);
        h_punta = k_arb;
    end
end
ganancia_arb = p_punta * ETA_BAT - Precio;          % EUR/MWh
arbitraje_ok = (h_punta >= 1) && (ganancia_arb > MARGEN_ARB);

%% Salidas
RefFC = 0; RefEl = 0; RefBat = 0; Compresor = 0;
DiscEl = [0 0 0]; DiscFC = [0 0 0];

Exced = PV - Carga;

comp_ok = (LOH_High < LOH_High_hi) && (LOH > LOH_reserva);
fac_comp = 0;
if comp_ok
    fac_comp = (LOH - LOH_reserva) / max(1e-6, (LOH_maxEL - LOH_reserva));
    fac_comp = max(0, min(1, fac_comp));
end
CompPermitido = PmaxComp * fac_comp;

%% Bloque 1 — reparto de potencia (gancho 1 en el excedente)
if Exced > 0
    PotLibre = Exced;

    if SOC < SOC_LOW,       wBat = 0.80; wEl = 0.20;
    elseif SOC < SOC_HIGH,  wBat = 0.60; wEl = 0.40;
    else,                   wBat = 0.30; wEl = 0.70;
    end

    % gancho 1: desplaza el reparto segun la tendencia prevista del excedente
    if pv_trend < 0
        delta = min(DELTA_W_MAX, wBat * 0.5) * min(1, abs(pv_trend) / max(PV, 1e-6));
    else
        delta = -min(DELTA_W_MAX, wEl * 0.5) * min(1, pv_trend / max(PV, 1e-6));
    end
    wEl  = max(0, min(1, wEl + delta));
    wBat = max(0, 1 - wEl);

    if SOC < SOC_MAX_PV
        PotBat = min(PmaxBat, min(wBat * PotLibre, PotLibre));
        RefBat = -PotBat;
        PotLibre = PotLibre - PotBat;
    end

    if (PotLibre > 0) && (LOH < LOH_maxEL)
        PotEl = min([PmaxEl, wEl * Exced, PotLibre]);
        RefEl = -PotEl;
        PotLibre = PotLibre - PotEl;
    end

    if (PotLibre > 0) && (LOH < LOH_maxEL)
        add = min(PmaxEl - abs(RefEl), PotLibre);
        if add > 0, RefEl = RefEl - add; PotLibre = PotLibre - add; end
    end
    if (PotLibre > 0) && (LOH_High < LOH_High_lo_on) && comp_ok
        add = min(CompPermitido, PotLibre);
        if add > 0, PotLibre = PotLibre - add; end
    end
    if (PotLibre > 0) && (SOC < SOC_MAX_PV)
        add = min(PmaxBat - abs(RefBat), PotLibre);
        if add > 0, RefBat = RefBat - add; PotLibre = PotLibre - add; end
    end
    if (PotLibre > 0) && comp_ok
        add = min(max(0, CompPermitido - Compresor), PotLibre);
        if add > 0, Compresor = Compresor + add; end
    end

elseif Exced < 0
    PotDef = -Exced;

    if SOC > SOC_MIN_DESC
        Pdesc = min(PotDef, PmaxBat);
        RefBat = Pdesc;
        PotDef = PotDef - Pdesc;
    end
    if PotDef > 0
        RefFC = min(PotDef, PmaxFC);
        PotDef = PotDef - RefFC;
    end
    if (LOH_High < LOH_High_crit) && comp_ok && (PotDef > 0)
        Compresor = min(CompPermitido, PotDef);
    end

    if LOH_High < LOH_High_lo_off
        if LOH > LOH_reserva, C_local_kg = C_comp_kg; else, C_local_kg = C_ELcomp_kg; end
        if C_local_kg <= H2_PRECIO_EXT_KG
            if LOH < LOH_maxEL, RefEl = min(RefEl, -PmaxEl); end
            if comp_ok, Compresor = max(Compresor, CompPermitido); end
        end
    end
end

%% Bloque 1B — gancho 2: arbitraje dimensionado
% (1) si el precio va a subir, mover excedente de la bateria al electrolizador
%     (suma constante: no importa de red)
if precio_sube && (Exced > 0) && (LOH < LOH_maxEL)
    P_el_act = abs(min(RefEl, 0));
    P_bat_act = abs(min(RefBat, 0));
    P_el_obj = min(0.5 * PmaxEl, Exced);
    if P_el_act < P_el_obj
        extra = min(P_el_obj - P_el_act, P_bat_act);
        if extra > 0
            RefEl  = -(P_el_act + extra);
            RefBat = -(P_bat_act - extra);
        end
    end
end

% (2) comprar de red la energia que falta para llegar a SOC_OBJ_ARB en la punta
if arbitraje_ok && (SOC < SOC_OBJ_ARB)
    E_falta_kWh = (SOC_OBJ_ARB - SOC) / 100 * CAP_BAT_kWh;
    P_arb       = E_falta_kWh / h_punta * 1000;      % kWh/h -> W
    P_arb       = min(P_arb, PmaxBat);
    RefBat = min(RefBat, -P_arb);                    % solo refuerza la carga
end

%% Bloque 2 — TMF + histeresis (igual que A)
[RefEl, EL_on, EL_t, EL_deb] = tmf_electrolizador( ...
    RefEl, EL_on, EL_t, EL_deb, TMF_s, Ts_s, P_EL_min_keep, thr_EL, DEB_on_s, LOH, LOH_maxEL);

[RefFC, FC_on, FC_t, FC_deb_on, FC_deb_off] = tmf_pila( ...
    RefFC, FC_on, FC_t, FC_deb_on, FC_deb_off, TMF_s, Ts_s, P_FC_min_keep, ...
    FC_thr_on, FC_thr_off, DEB_on_s, DEB_off_s);

%% Bloque 3 — maquina de estados Paro/Standby/Run (igual que A)
if EstEl(1) == 1
    DiscEl(1) = 1;
end
if EL_on && EstEl(2) == 1
    DiscEl(2) = 1;
end
if (~EL_on) && (EstEl(3) == 1)
    DiscEl(1) = 1;
    DiscEl(2) = 0;
end
if LOH >= LOH_maxEL || LOH_High >= LOH_High_hi
    RefEl = 0;
end

if EstFC(1) == 1
    DiscFC(1) = 1;
end
if FC_on && EstFC(2) == 1
    DiscFC(2) = 1;
end
if (~FC_on) && (EstFC(3) == 1)
    DiscFC(1) = 1;
    DiscFC(2) = 0;
end
if LOH_High <= LOH_min
    RefFC = 0;
end

end % fcn


%% Subfunciones TMF (identicas a A)
function [RefEl, EL_on, EL_t, EL_deb] = tmf_electrolizador( ...
    RefEl, EL_on, EL_t, EL_deb, TMF_s, Ts_s, P_min_keep, thr, DEB_on_s, LOH, LOH_maxEL)

want_on = (RefEl < -thr) && (LOH < LOH_maxEL);

if EL_on
    EL_t = EL_t + Ts_s;
    if ~want_on
        if EL_t < TMF_s
            RefEl = -max(P_min_keep, 0);
        else
            RefEl = 0; EL_on = false; EL_t = 0; EL_deb = 0;
        end
    end
else
    if want_on
        EL_deb = min(EL_deb + Ts_s, DEB_on_s);
        if EL_deb >= DEB_on_s
            EL_on = true; EL_t = 0;
            if RefEl > -P_min_keep, RefEl = -P_min_keep; end
        end
    else
        EL_deb = 0; RefEl = 0;
    end
end
end


function [RefFC, FC_on, FC_t, FC_deb_on, FC_deb_off] = tmf_pila( ...
    RefFC, FC_on, FC_t, FC_deb_on, FC_deb_off, TMF_s, Ts_s, P_min_keep, ...
    thr_on, thr_off, DEB_on_s, DEB_off_s)

want_on_now  = (RefFC > thr_on);
want_off_now = (RefFC < thr_off);

if FC_on
    FC_t = FC_t + Ts_s;
    if want_off_now
        FC_deb_off = min(FC_deb_off + Ts_s, DEB_off_s);
    else
        FC_deb_off = 0;
    end
    if FC_deb_off >= DEB_off_s
        if FC_t < TMF_s
            RefFC = max(P_min_keep, 0);
        else
            RefFC = 0; FC_on = false; FC_t = 0; FC_deb_on = 0; FC_deb_off = 0;
        end
    else
        FC_deb_on = 0;
    end
else
    if want_on_now
        FC_deb_on = min(FC_deb_on + Ts_s, DEB_on_s);
    else
        FC_deb_on = 0; RefFC = 0;
    end
    if FC_deb_on >= DEB_on_s
        FC_on = true; FC_t = 0; FC_deb_off = 0;
        if RefFC < P_min_keep, RefFC = P_min_keep; end
    end
end
end

== stateflow chart OASIS/PEM Fuel Cell/Chart ==
  settings: initializeOutput=1
  state EOFF1 [commented out]
  state Trans1 [commented out]
  state StandBy [commented out]
  state Trans2 [commented out]
  state Run [commented out]
  state Standby
    P_out=CRampa(P_ref,1);
    P_out=0;
    EOff=0;
    ESBy=1;
    ERun=0;
  state EOFF
    P_out=0;
    EOff=1;
    ESBy=0;
    ERun=0;
  state Trans3
    P_out=0;
    EOff=1;
    ESBy=1;
    ERun=0;
  state Trans4
    P_out=CRampa(P_ref,0);
    EOff=0;
    ESBy=1;
    ERun=1;
  state Run1
    P_out=P_ref;
    EOff=0;
    ESBy=0;
    ERun=1;
  state PSal = CRampa(Ref,Reset) [function]
  (default) -> EOFF1 [commented out]
  Trans2 -> Run [commented out] : after(180,sec)
  EOFF1 -> Trans1 [commented out] : [Stby==1]
  StandBy -> Trans2 [commented out] : [Run==1]
  Trans1 -> StandBy [commented out] : after(380,sec)
  Run -> StandBy [commented out] : [Stby==1]
  (default) -> EOFF
  EOFF -> Trans3 : [Stby==1]
  Trans3 -> Standby : after(380,sec)
  Standby -> Trans4 [order 1] : [Run==1]
  Trans4 -> Run1 : after(180,sec)
  Standby -> EOFF [order 2] : [OFF==1]
  Run1 -> Standby : [Stby==1]
  data: sf_internal_action_state_placeholder_data local double size=1 =0; sf_internal_action_state_placeholder_data local double size=1 =0; sf_internal_action_state_placeholder_data local double size=1 =0; sf_internal_action_state_placeholder_data local double size=1 =0; sf_internal_action_state_placeholder_data local double size=1 =0; Ref function_input double size=1; PSal function_output; Reset function_input double size=1; P_ref input; P_out output; Stby input; EOff output; ESBy output; ERun output; Run input; OFF input
